simulink model "AircraftDynamicSimNonLinear"  (R2024a)
settings: Solver=ode4  StartTime=0.0  StopTime=200  FixedStep=0.01  RelTol=1e-3  EnableMultiTasking=on
undefined symbols (not defined in the file): CG_mac, Mass_kg
libraries: AircraftSixDOFModel x1
settings Model: Creator=mahariansyah  LastModifiedBy=mahariansyah
settings DataIOCC: ExternalInput=getinputstruct(opreport_climb)  InitialState=getstatestruct(opreport_cruise)

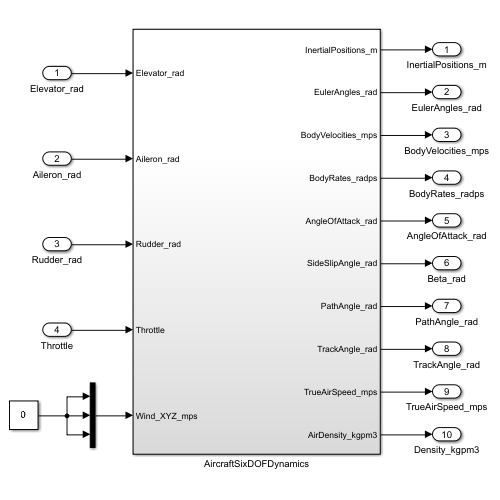
[thumbnail: Simulink's stored preview of the top-level diagram]
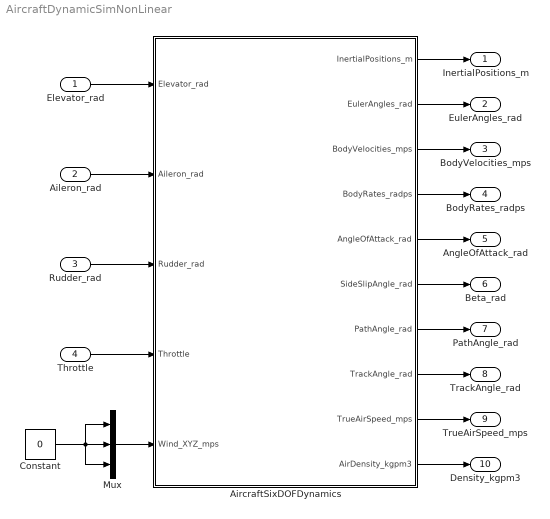
== system AircraftDynamicSimNonLinear ==
  Elevator_rad : Inport
  Aileron_rad : Inport  Port=2
  Rudder_rad : Inport  Port=3
  Throttle : Inport  Port=4
  AircraftSixDOFDynamics : Subsystem
  Constant : Constant  Value=0
  Mux : Mux  Inputs=3
  InertialPositions_m : Outport
  EulerAngles_rad : Outport  Port=2
  BodyVelocities_mps : Outport  Port=3
  BodyRates_radps : Outport  Port=4
  AngleOfAttack_rad : Outport  Port=5
  Beta_rad : Outport  Port=6
  PathAngle_rad : Outport  Port=7
  TrackAngle_rad : Outport  Port=8
  TrueAirSpeed_mps : Outport  Port=9
  Density_kgpm3 : Outport  Port=10
  wires:
  AircraftSixDOFDynamics/5(AngleOfAttack_rad) -> AngleOfAttack_rad/1
  AircraftSixDOFDynamics/6(SideSlipAngle_rad) -> Beta_rad/1
  AircraftSixDOFDynamics/3(BodyVelocities_mps) -> BodyVelocities_mps/1
  AircraftSixDOFDynamics/4(BodyRates_radps) -> BodyRates_radps/1
  AircraftSixDOFDynamics/2(EulerAngles_rad) -> EulerAngles_rad/1
  AircraftSixDOFDynamics/7(PathAngle_rad) -> PathAngle_rad/1
  AircraftSixDOFDynamics/1(InertialPositions_m) -> InertialPositions_m/1
  Throttle/1 -> AircraftSixDOFDynamics/4(Throttle)
  Elevator_rad/1 -> AircraftSixDOFDynamics/1(Elevator_rad)
  Mux/1 -> AircraftSixDOFDynamics/5(Wind_XYZ_mps)
  Constant/1 -> Mux/1, Mux/3, Mux/2
  AircraftSixDOFDynamics/9(TrueAirSpeed_mps) -> TrueAirSpeed_mps/1
  AircraftSixDOFDynamics/10(AirDensity_kgpm3) -> Density_kgpm3/1
  Aileron_rad/1 -> AircraftSixDOFDynamics/2(Aileron_rad)
  Rudder_rad/1 -> AircraftSixDOFDynamics/3(Rudder_rad)
  AircraftSixDOFDynamics/8(TrackAngle_rad) -> TrackAngle_rad/1

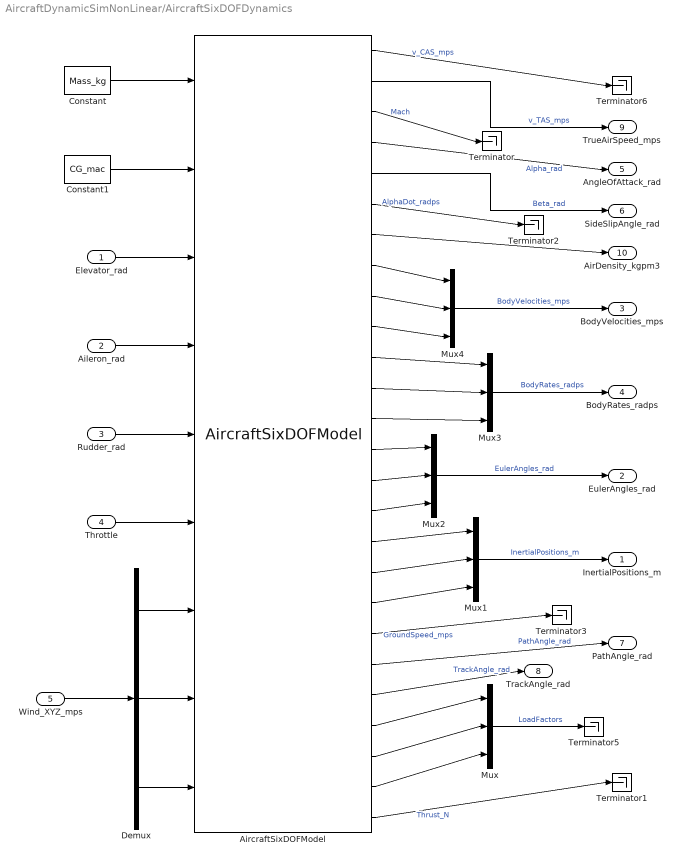
== system AircraftDynamicSimNonLinear/AircraftSixDOFDynamics ==
  Elevator_rad : Inport
  Aileron_rad : Inport  Port=2
  Rudder_rad : Inport  Port=3
  Throttle : Inport  Port=4
  Wind_XYZ_mps : Inport  Port=5
  AircraftSixDOFModel : AircraftSixDOFModel/AircraftSixDOFModel  SystemSampleTime=-1  VariantActivationTime=update diagram  AllowFlexibleInterface=on  Latency=0  AutoFrameSizeCalculation=off
  Constant : Constant  Value=Mass_kg
  Constant1 : Constant  Value=CG_mac
  Demux : Demux  Outputs=3
  Mux{,1..4} (5 alike) : Mux  Inputs=3
  Terminator{,1..3,5..6} (6 alike) : Terminator
  InertialPositions_m : Outport
  EulerAngles_rad : Outport  Port=2
  BodyVelocities_mps : Outport  Port=3
  BodyRates_radps : Outport  Port=4
  AngleOfAttack_rad : Outport  Port=5
  SideSlipAngle_rad : Outport  Port=6
  PathAngle_rad : Outport  Port=7
  TrackAngle_rad : Outport  Port=8
  TrueAirSpeed_mps : Outport  Port=9
  AirDensity_kgpm3 : Outport  Port=10
  wires:
  AircraftSixDOFModel/6 -> Terminator2/1  "AlphaDot_radps"
  Mux4/1 -> BodyVelocities_mps/1  "BodyVelocities_mps"
  Wind_XYZ_mps/1 -> Demux/1
  Rudder_rad/1 -> AircraftSixDOFModel/5
  Elevator_rad/1 -> AircraftSixDOFModel/3
  Aileron_rad/1 -> AircraftSixDOFModel/4
  Constant1/1 -> AircraftSixDOFModel/2
  AircraftSixDOFModel/3 -> Terminator/1  "Mach"
  Demux/1 -> AircraftSixDOFModel/7
  Demux/2 -> AircraftSixDOFModel/8
  Mux2/1 -> EulerAngles_rad/1  "EulerAngles_rad"
  AircraftSixDOFModel/4 -> AngleOfAttack_rad/1  "Alpha_rad"
  Mux3/1 -> BodyRates_radps/1  "BodyRates_radps"
  AircraftSixDOFModel/2 -> TrueAirSpeed_mps/1  "v_TAS_mps"
  Mux1/1 -> InertialPositions_m/1  "InertialPositions_m"
  Throttle/1 -> AircraftSixDOFModel/6
  AircraftSixDOFModel/1 -> Terminator6/1  "v_CAS_mps"
  Constant/1 -> AircraftSixDOFModel/1
  Demux/3 -> AircraftSixDOFModel/9
  AircraftSixDOFModel/5 -> SideSlipAngle_rad/1  "Beta_rad"
  Mux/1 -> Terminator5/1  "LoadFactors"
  AircraftSixDOFModel/8 -> Mux4/1
  AircraftSixDOFModel/9 -> Mux4/2
  AircraftSixDOFModel/10 -> Mux4/3
  AircraftSixDOFModel/11 -> Mux3/1
  AircraftSixDOFModel/12 -> Mux3/2
  AircraftSixDOFModel/13 -> Mux3/3
  AircraftSixDOFModel/14 -> Mux2/1
  AircraftSixDOFModel/15 -> Mux2/2
  AircraftSixDOFModel/16 -> Mux2/3
  AircraftSixDOFModel/17 -> Mux1/1
  AircraftSixDOFModel/18 -> Mux1/2
  AircraftSixDOFModel/19 -> Mux1/3
  AircraftSixDOFModel/26 -> Terminator1/1  "Thrust_N"
  AircraftSixDOFModel/23 -> Mux/1
  AircraftSixDOFModel/24 -> Mux/2
  AircraftSixDOFModel/25 -> Mux/3
  AircraftSixDOFModel/22 -> TrackAngle_rad/1  "TrackAngle_rad"
  AircraftSixDOFModel/21 -> PathAngle_rad/1  "PathAngle_rad"
  AircraftSixDOFModel/20 -> Terminator3/1  "GroundSpeed_mps"
  AircraftSixDOFModel/7 -> AirDensity_kgpm3/1
